simulink model "GreenCraneSimulator"  (R2021b)
settings: Solver=ode23  StartTime=0.0  StopTime=25  FixedStep=0.0001  RelTol=1e-3
values from neighbouring files (symbols this model uses):
  Annulus_area = Bore_area-Rod_area    (= 2356.19449019)    [param.m]
  beta_F = 12000e5    (= 1200000000)    [param.m]
  Bore_area = pi/4*Bore_diameter^2    (= 3318.30724035)    [param.m]
  cyl_c_end = 9e8    (= 900000000)    [param.m]
  cyl_c_visc = 1500    [param.m]
  cyl_CH_stat = 1/50    (= 0.02)    [param.m]
  cyl_F_coul = 75    [param.m]
  cyl_FH_stat = 500    [param.m]
  cyl_gamma = 250    [param.m]
  cyl_k_end = 6e9    (= 6000000000)    [param.m]
  dr_dcv = 0.7    [param.m]
  Eff_Bulk_On = 1    [param.m]
  eta_air = 0.7e-2    (= 0.007)    [param.m]
  k_cv = 15    [param.m]
  k_DCV_PA = 7.9    [param.m]
  k_DCV_PB = 7.78    [param.m]
  k_DCV_T = 7.9    [param.m]
  k_ocv = 15    [param.m]
  K_oil = 12000    [param.m]
  k_tanh = 0.005    [param.m]
  kappa_air = 1.4    [param.m]
  mu_ocv = 3    [param.m]
  OL_pa = -0.114    [param.m]
  OL_pb = 0.114    [param.m]
  p0_A = 70.5441    [param.m]
  p0_A1 = 0.99958    [param.m]
  p0_B = 1.1    [param.m]
  p_cv_fo = 1    [param.m]
  p_cv_set = 2.8    [param.m]
  p_ocv_fo = 350    [param.m]
  p_ocv_set = 150    [param.m]
  p_pc_set = 7    [param.m]
  p_R = 1.1    [param.m]
  p_S = 180    [param.m]
  patm = 1.013e5    (= 101300)    [param.m]
  Stroke = 500    [param.m]
  tau_ocv = 0.0889*0+0.055    (= 0.055)    [param.m]
  tau_pc = 0.009    [param.m]
  tCycle = 0.01    [param.m]
  UL_at = -0.05    [param.m]
  UL_bt = 0.05    [param.m]
  V_CH_A = 1.0e-03    (= 0.001)    [param.m]
  V_CH_A1 = 0.1e-03    (= 0.0001)    [param.m]
  V_CH_B = 1.25e-03    (= 0.00125)    [param.m]
  v_cyl_0 = 0    [param.m]
  wn_dcv = 30    [param.m]
  x_cyl_0 = 0.05    [param.m]
undefined symbols (not defined in the file or in its folder): DiscIntNeverNeededParam, X, Y, Z
libraries: sm_lib x25, nesl_utility x4, simulink x1
(part 2 of 2)

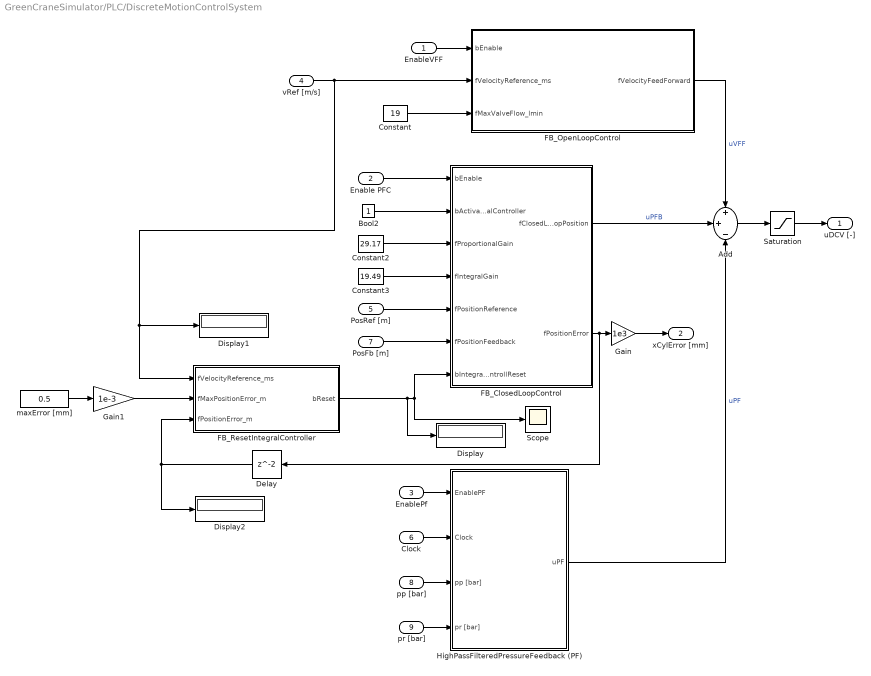
== system GreenCraneSimulator/PLC/DiscreteMotionControlSystem ==
  EnableVFF : Inport
  Enable PFC : Inport  Port=2
  EnablePf : Inport  Port=3
  vRef [m/s] : Inport  Port=4
  PosRef [m] : Inport  Port=5
  Clock : Inport  Port=6
  PosFb [m] : Inport  Port=7
  pp [bar] : Inport  Port=8
  pr [bar] : Inport  Port=9
  Add : Sum  Inputs=++-
  Bool2 : Constant  OutDataTypeStr=boolean
  Constant : Constant  Value=19
  Constant2 : Constant  Value=29.17
  Constant3 : Constant  Value=19.49
  Delay : Delay
  Display : Display
  Display1 : Display
  Display2 : Display
  FB_ClosedLoopControl : Subsystem  TreatAsAtomicUnit=on
  FB_OpenLoopControl : Subsystem  TreatAsAtomicUnit=on
  FB_ResetIntegralController : Subsystem  TreatAsAtomicUnit=on
  Gain : Gain  Gain=1e3
  Gain1 : Gain  Gain=1e-3
  HighPassFilteredPressureFeedback (PF) : Subsystem  TreatAsAtomicUnit=on  SystemSampleTime=tCycle
  Saturation : Saturate  UpperLimit=1  LowerLimit=-1
  Scope : Scope
  maxError [mm] : Constant  Value=0.5
  uDCV [-] : Outport
  xCylError [mm] : Outport  Port=2
  wires:
  Constant2/1 -> FB_ClosedLoopControl/3(fProportionalGain)
  Enable PFC/1 -> FB_ClosedLoopControl/1(bEnable)
  Constant3/1 -> FB_ClosedLoopControl/4(fIntegralGain)
  EnableVFF/1 -> FB_OpenLoopControl/1(bEnable)
  Bool2/1 -> FB_ClosedLoopControl/2(bActivateIntegralController)
  FB_ClosedLoopControl/2(fPositionError) -> Delay/1, Gain/1
  HighPassFilteredPressureFeedback (PF)/1(uPF) -> Add/3  "uPF"
  Constant/1 -> FB_OpenLoopControl/3(fMaxValveFlow_lmin)
  FB_OpenLoopControl/1(fVelocityFeedForward) -> Add/1  "uVFF"
  FB_ClosedLoopControl/1(fClosedLoopPosition) -> Add/2  "uPFB"
  PosFb [m]/1 -> FB_ClosedLoopControl/6(fPositionFeedback)
  PosRef [m]/1 -> FB_ClosedLoopControl/5(fPositionReference)
  EnablePf/1 -> HighPassFilteredPressureFeedback (PF)/1(EnablePF)
  Clock/1 -> HighPassFilteredPressureFeedback (PF)/2(Clock)
  pp [bar]/1 -> HighPassFilteredPressureFeedback (PF)/3(pp [bar])
  pr [bar]/1 -> HighPassFilteredPressureFeedback (PF)/4(pr [bar])
  Add/1 -> Saturation/1
  Gain/1 -> xCylError [mm]/1
  maxError [mm]/1 -> Gain1/1
  Saturation/1 -> uDCV [-]/1
  FB_ResetIntegralController/1(bReset) -> Display/1, FB_ClosedLoopControl/7(bIntegralControllReset), Scope/1
  Delay/1 -> FB_ResetIntegralController/3(fPositionError_m), Display2/1
  Gain1/1 -> FB_ResetIntegralController/2(fMaxPositionError_m)
  vRef [m/s]/1 -> FB_OpenLoopControl/2(fVelocityReference_ms), FB_ResetIntegralController/1(fVelocityReference_ms), Display1/1

== system GreenCraneSimulator/PLC/MotionRefSelector ==
  Auto [1] / Man [0] : Inport  OutDataTypeStr=boolean
  xCylRefGen [m] : Inport  Port=2
  vCylRefGen [m] : Inport  Port=3
  vCylJoy [m/s] : Inport  Port=4
  Data Type Conversion : DataTypeConversion  OutDataTypeStr=boolean
  Data Type Conversion1 : DataTypeConversion  OutDataTypeStr=boolean
  MATLAB Function : MATLAB Function  TreatAsAtomicUnit=on
  VFF Enable : Outport  OutDataTypeStr=boolean
  PFC Enable : Outport  Port=2  OutDataTypeStr=boolean
  vCylRef [m/s] : Outport  Port=3
  xCylRef [m] : Outport  Port=4
  wires:
  Auto [1] / Man [0]/1 -> MATLAB Function/1(AutoMode)
  vCylJoy [m/s]/1 -> MATLAB Function/4(VelRefMan)
  xCylRefGen [m]/1 -> MATLAB Function/3(PosRefAuto)
  vCylRefGen [m]/1 -> MATLAB Function/2(VelRefAuto)
  MATLAB Function/1(VelRef) -> vCylRef [m/s]/1
  MATLAB Function/2(PosRef) -> xCylRef [m]/1
  MATLAB Function/3(VFF) -> Data Type Conversion1/1
  MATLAB Function/4(PFC) -> Data Type Conversion/1
  Data Type Conversion/1 -> PFC Enable/1
  Data Type Conversion1/1 -> VFF Enable/1

== system GreenCraneSimulator/PLC/MotionReferenceTime ==
  <StartAuto> : Inport
  <StopAuto> : Inport  Port=2
  Constant : Constant
  Discrete-Time Integrator : DiscreteIntegrator  SampleTime=-1  ICPrevOutput=DiscIntNeverNeededParam  ICPrevScaledInput=DiscIntNeverNeededParam
  MATLAB Function : MATLAB Function  TreatAsAtomicUnit=on
  Time : Outport
  wires:
  <StartAuto>/1 -> MATLAB Function/1(StartClock)
  <StopAuto>/1 -> MATLAB Function/2(StopClock)
  Constant/1 -> Discrete-Time Integrator/1
  MATLAB Function/1(Time) -> Time/1
  Discrete-Time Integrator/1 -> MATLAB Function/3(Clock)

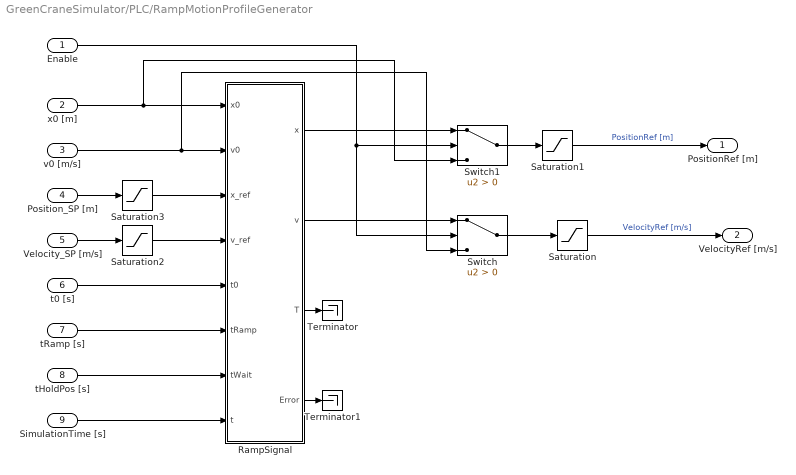
== system GreenCraneSimulator/PLC/RampMotionProfileGenerator ==
  Enable : Inport  OutDataTypeStr=boolean
  x0 [m] : Inport  Port=2  OutDataTypeStr=double
  v0 [m/s] : Inport  Port=3  OutDataTypeStr=double
  Position_SP [m] : Inport  Port=4  OutDataTypeStr=double
  "Velocity_SP [m/s] " : Inport  Port=5  OutDataTypeStr=double
  t0 [s] : Inport  Port=6  OutDataTypeStr=double
  tRamp [s] : Inport  Port=7  OutDataTypeStr=double
  tHoldPos [s] : Inport  Port=8  OutDataTypeStr=double
  SimulationTime [s] : Inport  Port=9  OutDataTypeStr=double
  RampSignal : MATLAB Function  TreatAsAtomicUnit=on
  Saturation : Saturate  UpperLimit=150  LowerLimit=-150
  Saturation1 : Saturate  UpperLimit=500  LowerLimit=0
  Saturation2 : Saturate  UpperLimit=0.120  LowerLimit=0
  Saturation3 : Saturate  LowerLimit=0
  Switch : Switch  Criteria=u2 > Threshold
  Switch1 : Switch  Criteria=u2 > Threshold
  Terminator : Terminator
  Terminator1 : Terminator
  "PositionRef [m] " : Outport  VectorParamsAs1DForOutWhenUnconnected=off
  VelocityRef [m/s] : Outport  Port=2  VectorParamsAs1DForOutWhenUnconnected=off
  wires:
  SimulationTime [s]/1 -> RampSignal/8(t)
  RampSignal/2(v) -> Switch/1
  Switch/1 -> Saturation/1
  v0 [m/s]/1 -> RampSignal/2(v0), Switch/3
  t0 [s]/1 -> RampSignal/5(t0)
  Position_SP [m]/1 -> Saturation3/1
  tHoldPos [s]/1 -> RampSignal/7(tWait)
  "Velocity_SP [m/s] "/1 -> Saturation2/1
  RampSignal/1(x) -> Switch1/1
  Enable/1 -> Switch/2, Switch1/2
  x0 [m]/1 -> Switch1/3, RampSignal/1(x0)
  Switch1/1 -> Saturation1/1
  Saturation2/1 -> RampSignal/4(v_ref)
  Saturation3/1 -> RampSignal/3(x_ref)
  tRamp [s]/1 -> RampSignal/6(tRamp)
  RampSignal/3(T) -> Terminator/1
  RampSignal/4(Error) -> Terminator1/1
  Saturation1/1 -> "PositionRef [m] "/1  "PositionRef [m]"
  Saturation/1 -> VelocityRef [m/s]/1  "VelocityRef [m/s]"

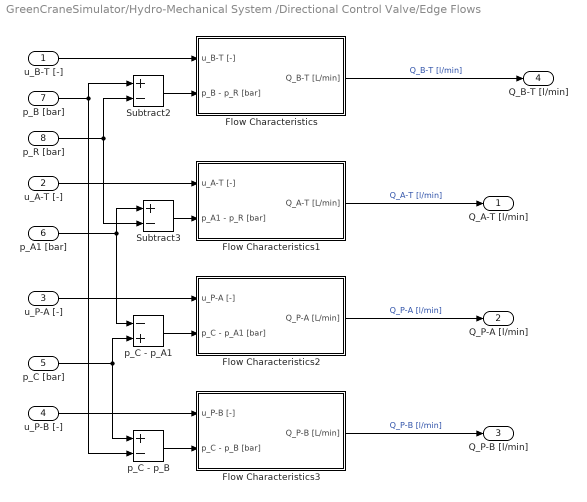
== system GreenCraneSimulator/Hydro-Mechanical System /Directional Control Valve/Edge Flows ==
  u_B-T [-] : Inport
  u_A-T [-] : Inport  Port=2
  u_P-A [-] : Inport  Port=3
  u_P-B [-] : Inport  Port=4
  p_C [bar] : Inport  Port=5
  p_A1 [bar] : Inport  Port=6
  p_B [bar] : Inport  Port=7
  p_R [bar] : Inport  Port=8
  Flow Characteristics : Subsystem
  Flow Characteristics1 : Subsystem
  Flow Characteristics2 : Subsystem
  Flow Characteristics3 : Subsystem
  Subtract2 : Sum  Inputs=+-
  Subtract3 : Sum  Inputs=+-
  p_C - p_A1 : Sum  Inputs=-+
  p_C - p_B : Sum  Inputs=+-
  Q_A-T [l/min] : Outport  VectorParamsAs1DForOutWhenUnconnected=off
  Q_P-A [l/min] : Outport  Port=2  VectorParamsAs1DForOutWhenUnconnected=off
  Q_P-B [l/min] : Outport  Port=3  VectorParamsAs1DForOutWhenUnconnected=off
  Q_B-T [l/min] : Outport  Port=4  VectorParamsAs1DForOutWhenUnconnected=off
  wires:
  p_C [bar]/1 -> p_C - p_A1/2, p_C - p_B/1
  u_A-T [-]/1 -> Flow Characteristics1/1(u_A-T [-])
  p_A1 [bar]/1 -> Subtract3/1, p_C - p_A1/1
  p_B [bar]/1 -> Subtract2/1, p_C - p_B/2
  p_C - p_B/1 -> Flow Characteristics3/2(p_C - p_B [bar])
  u_P-A [-]/1 -> Flow Characteristics2/1(u_P-A [-])
  p_C - p_A1/1 -> Flow Characteristics2/2(p_C - p_A1 [bar])
  u_P-B [-]/1 -> Flow Characteristics3/1(u_P-B [-])
  p_R [bar]/1 -> Subtract3/2, Subtract2/2
  Flow Characteristics1/1(Q_A-T [L/min]) -> Q_A-T [l/min]/1  "Q_A-T [l/min]"
  Flow Characteristics/1(Q_B-T [L/min]) -> Q_B-T [l/min]/1  "Q_B-T [l/min]"
  Flow Characteristics3/1(Q_P-B [L/min]) -> Q_P-B [l/min]/1  "Q_P-B [l/min]"
  Flow Characteristics2/1(Q_P-A [L/min]) -> Q_P-A [l/min]/1  "Q_P-A [l/min]"
  Subtract2/1 -> Flow Characteristics/2(p_B - p_R [bar])
  u_B-T [-]/1 -> Flow Characteristics/1(u_B-T [-])
  Subtract3/1 -> Flow Characteristics1/2(p_A1 - p_R [bar])

== system GreenCraneSimulator/Hydro-Mechanical System /Directional Control Valve/Edge Openings ==
  u_dcv [-] : Inport
  Edge A-T : Subsystem
  Edge B-T : Subsystem
  Edge P-A : Subsystem
  Edge P-B : Subsystem
  u_B-T [-] : Outport  VectorParamsAs1DForOutWhenUnconnected=off
  u_A-T [-] : Outport  Port=2  VectorParamsAs1DForOutWhenUnconnected=off
  u_P-A [-] : Outport  Port=3  VectorParamsAs1DForOutWhenUnconnected=off
  u_P-B [-] : Outport  Port=4  VectorParamsAs1DForOutWhenUnconnected=off
  wires:
  Edge A-T/1(u_A-T [-]) -> u_A-T [-]/1  "u_A-T [-]"
  Edge B-T/1(u_B-T [-]) -> u_B-T [-]/1  "u_B-T [-]"
  u_dcv [-]/1 -> Edge P-A/1(u_dcv [-]), Edge P-B/1(u_dcv [-]), Edge A-T/1(u_dcv [-]), Edge B-T/1(u_dcv [-])  "[-]"
  Edge P-A/1(u_P-A [-]) -> u_P-A [-]/1  "u_P-A [-]"
  Edge P-B/1(u_P-B [-]) -> u_P-B [-]/1  "u_P-B [-]"

== system GreenCraneSimulator/Hydro-Mechanical System /Directional Control Valve/Load-Sensing Pressure ==
  pB : Inport
  pA1 : Inport  Port=2
  uDCV : Inport  Port=3
  Constant : Constant  Value=0
  Switch : Switch  Criteria=u2 ~= 0
  Switch1 : Switch  Criteria=u2 > Threshold
  pLS : Outport  VectorParamsAs1DForOutWhenUnconnected=off
  wires:
  pA1/1 -> Switch1/3
  Constant/1 -> Switch/3
  Switch1/1 -> Switch/1
  Switch/1 -> pLS/1
  uDCV/1 -> Switch1/2, Switch/2
  pB/1 -> Switch1/1

== system GreenCraneSimulator/Hydro-Mechanical System /Directional Control Valve/Valve Dynamics ==
  note: 2nd order TF for
      | DCV dynamics
  u_dcv_ref [-] : Inport
  2nd order TF : TransferFcn  Denominator="[1/(wn_dcv^2) 2*dr_dcv/wn_dcv  1]"
  u_dcv [-] : Outport  VectorParamsAs1DForOutWhenUnconnected=off
  wires:
  u_dcv_ref [-]/1 -> 2nd order TF/1  "u_dcv_ref [-]"
  2nd order TF/1 -> u_dcv [-]/1  "u_dcv [-]"

== system GreenCraneSimulator/Hydro-Mechanical System /Over-Centre Valve/Capasitance ==
  Bulk Modulus : Subsystem
  Constant : Constant  Value=V_CH_A1
  Divide : Product  Inputs=*/
  "CH_A1 " : Outport  VectorParamsAs1DForOutWhenUnconnected=off
  wires:
  Bulk Modulus/1(K_oil) -> Divide/2  "[bar]"
  Constant/1 -> Divide/1  "[m^3]"
  Divide/1 -> "CH_A1 "/1

== system GreenCraneSimulator/Hydro-Mechanical System /Over-Centre Valve/Check Valve ==
  p_A [bar] : Inport
  p_A1 [bar] : Inport  Port=2
  Abs : Abs  ZeroCross=off
  Constant : Constant  Value=k_cv
  Product : Product  Inputs=****
  Saturation : Saturate  UpperLimit=1  LowerLimit=0  ZeroCross=off
  Sign : Subsystem
  Sqrt : Sqrt  SaturateOnIntegerOverflow=on
  Sum : Sum  Inputs=+-
  Sum1 : Sum  Inputs=+-
  division by p_cv_fo : Gain  Gain=1/p_cv_fo
  p_cv_set [bar] : Constant  Value=p_cv_set
  Q_cv [l/min]1 : Outport  VectorParamsAs1DForOutWhenUnconnected=off
  wires:
  p_cv_set [bar]/1 -> Sum1/2
  Sum/1 -> Abs/1, Sum1/1, Sign/1(In)  "p2-p3 [bar]"
  p_A [bar]/1 -> Sum/2
  p_A1 [bar]/1 -> Sum/1
  division by p_cv_fo/1 -> Saturation/1  "u_cv [-]"
  Sum1/1 -> division by p_cv_fo/1
  Constant/1 -> Product/1  "[l/min/bar^0.5]"
  Sqrt/1 -> Product/2  "[bar^0.5]"
  Sign/1(Out) -> Product/4
  Saturation/1 -> Product/3  "[-]"
  Abs/1 -> Sqrt/1
  Product/1 -> Q_cv [l/min]1/1

== system GreenCraneSimulator/Hydro-Mechanical System /Over-Centre Valve/Over-Centre Valve ==
  u_ocv [-] : Inport
  p_A [bar] : Inport  Port=2
  p_A1 [bar] : Inport  Port=3
  Abs : Abs  ZeroCross=off
  Product : Product  Inputs=****
  Sign : Subsystem
  Sqrt : Sqrt  SaturateOnIntegerOverflow=on
  k_ocv [l/min/bar^0.5] : Constant  Value=k_ocv
  p3-p2 : Sum  Inputs=+-
  "[l/min]" : Outport  VectorParamsAs1DForOutWhenUnconnected=off
  wires:
  k_ocv [l/min/bar^0.5]/1 -> Product/3
  p3-p2/1 -> Sign/1(In), Abs/1  "p3-p2 [bar]"
  Sqrt/1 -> Product/2  "[bar^0.5]"
  Sign/1(Out) -> Product/4
  p_A1 [bar]/1 -> p3-p2/2
  p_A [bar]/1 -> p3-p2/1
  Abs/1 -> Sqrt/1
  u_ocv [-]/1 -> Product/1  "[-]"
  Product/1 -> "[l/min]"/1

== system GreenCraneSimulator/Hydro-Mechanical System /Over-Centre Valve/Pressure Equillibrium ==
  p_B [bar] : Inport
  p_A [bar] : Inport  Port=2
  Division by p_ocv_fo [bar] : Gain  Gain=1/p_ocv_fo
  Pilot ratio [-] : Gain  Gain=mu_ocv
  Saturation : Saturate  UpperLimit=1  LowerLimit=0  ZeroCross=off
  Sum : Sum  Inputs=++-
  Valve Dynamics : TransferFcn  Denominator=[tau_ocv 1]
  p_ocv_set [bar] : Constant  Value=p_ocv_set
  u_ocv [-] : Outport  VectorParamsAs1DForOutWhenUnconnected=off
  wires:
  Sum/1 -> Division by p_ocv_fo [bar]/1  "[bar]"
  Pilot ratio [-]/1 -> Sum/1
  p_ocv_set [bar]/1 -> Sum/3
  p_B [bar]/1 -> Pilot ratio [-]/1
  p_A [bar]/1 -> Sum/2
  Valve Dynamics/1 -> u_ocv [-]/1  "[-]"
  Division by p_ocv_fo [bar]/1 -> Saturation/1  "u_ocv_ref [-]"
  Saturation/1 -> Valve Dynamics/1

== system GreenCraneSimulator/Hydro-Mechanical System /Subsystem/CH Bore Side ==
  x [m] : Inport
  Bulk Modulus : Subsystem
  Constant4 : Constant  Value=V_CH_A
  Divide2 : Product  Inputs=*/
  Gain1 : Gain  Gain=Bore_area
  Gain2 : Gain  Gain=1/(10)^9
  Gain3 : Gain  Gain=1000
  Scope : Scope
  Sum3 : Sum
  CH_A : Outport  VectorParamsAs1DForOutWhenUnconnected=off
  wires:
  Sum3/1 -> Divide2/1  "[m^3]"
  x [m]/1 -> Gain3/1
  Constant4/1 -> Sum3/1  "[m^3]"
  Gain1/1 -> Gain2/1  "[mm^3]"
  Gain3/1 -> Gain1/1  "[mm]"
  Gain2/1 -> Scope/1, Sum3/2  "[m^3]"
  Divide2/1 -> CH_A/1
  Bulk Modulus/1(K_oil) -> Divide2/2  "[bar]"

== system GreenCraneSimulator/Hydro-Mechanical System /Subsystem/CH Rod Side ==
  x [m] : Inport
  Bulk Modulus : Subsystem
  Constant1 : Constant  Value=Stroke
  Constant4 : Constant  Value=V_CH_B
  Divide2 : Product  Inputs=*/
  Gain1 : Gain  Gain=Annulus_area
  Gain2 : Gain  Gain=1/(10)^9
  Gain4 : Gain  Gain=1000
  Scope : Scope
  Sum2 : Sum  Inputs=+-
  Sum3 : Sum
  CH_B : Outport  VectorParamsAs1DForOutWhenUnconnected=off
  wires:
  Sum3/1 -> Divide2/1  "[m^3]"
  Constant1/1 -> Sum2/1  "[mm]"
  x [m]/1 -> Gain4/1
  Sum2/1 -> Gain1/1
  Constant4/1 -> Sum3/1  "[m^3]"
  Gain1/1 -> Gain2/1  "[mm^3]"
  Gain4/1 -> Sum2/2  "[mm]"
  Gain2/1 -> Sum3/2, Scope/1  "[m^3]"
  Divide2/1 -> CH_B/1
  Bulk Modulus/1(K_oil) -> Divide2/2

== system GreenCraneSimulator/Hydro-Mechanical System /Subsystem/Cylinder forces ==
  v_cyl [m/s] : Inport
  F_hyd [N] : Inport  Port=2
  x _cyl [m] : Inport  Port=3
  Add : Sum  Inputs=+-+-
  Lower Stroke Limit : Subsystem
  Stribeck Friction1 : Subsystem
  Upper Stroke Limit : Subsystem
  F_piston [N] : Outport  VectorParamsAs1DForOutWhenUnconnected=off
  wires:
  Lower Stroke Limit/1(F_cyl_contact [N]) -> Add/3
  Upper Stroke Limit/1(F_cyl_contact [N]) -> Add/2
  x _cyl [m]/1 -> Upper Stroke Limit/1(x_cyl [m]), Lower Stroke Limit/1(x_cyl [m])
  Add/1 -> F_piston [N]/1  "Bm_Cyl_F"
  v_cyl [m/s]/1 -> Stribeck Friction1/1(v_cyl [m/s]), Lower Stroke Limit/2(v_cyl [m]), Upper Stroke Limit/2(v_cyl [m/s])
  Stribeck Friction1/1(F [N]) -> Add/4
  F_hyd [N]/1 -> Add/1

== system GreenCraneSimulator/PC | Ubuntu | ROS2/Green Crane | Visualizer /Setup ==
  Mechanism Configuration1 : sm_lib/Utilities/Mechanism Configuration  UniformGravity=Constant  GravityVector=[0 0 -9.80665]  GravityUnits=m/s^2  LinearizationDelta=0.001  JointModeTransitionNonlinearIterations=2
  Solver Configuration : nesl_utility/Solver Configuration  PhysicalDomain=network_engine_domain  SubClassName=solver  LeftPortType=input  RightPortType=generic  Tones=[]  Harmonics=[]  SimulateNoise=off  Profile=off  UseLocalSampling=off  EnableSwitchedLinearOptims=on  FrequencyDomain=off  UseCCode=off  RelTol=0.001  AbsTol=1e-06  MinStep=1e-09  ToWorkspace=off  RevertToSquareIcSolve=off  NumHomotopyIterations=100  PhasorMode=off  PhasorModeNumHarmonics=1  DoDC=off  ResidualTolerance=1e-09  UseLocalSolver=off  LocalSolverChoice=NE_BACKWARD_EULER_ADVANCER  LocalSolverSampleTime=0.001  DoFixedCost=off  MaxNonlinIter=3  MaxModeIter=2  ComputeImpulses=off  ImpulseIterations=2  LinearAlgebra=Sparse  EquationFormulation=NE_TIME_EF  DelaysMemoryBudget=1024  AutomaticFiltering=on  FilteringTimeConstant=0.001  PartitionStorageMethod=AS_NEEDED  PartitionMemoryBudget=1024  PartitionMethod=FAST
      settings: SourceProductBaseCode=PW,SS
  World Frame : sm_lib/Frames and Transforms/World Frame
  Origin : PMIOPort  Side=Right
  connections:
  Solver Configuration/RConn1 -- World Frame/RConn1 -- Mechanism Configuration1/RConn1 -- Origin/RConn1

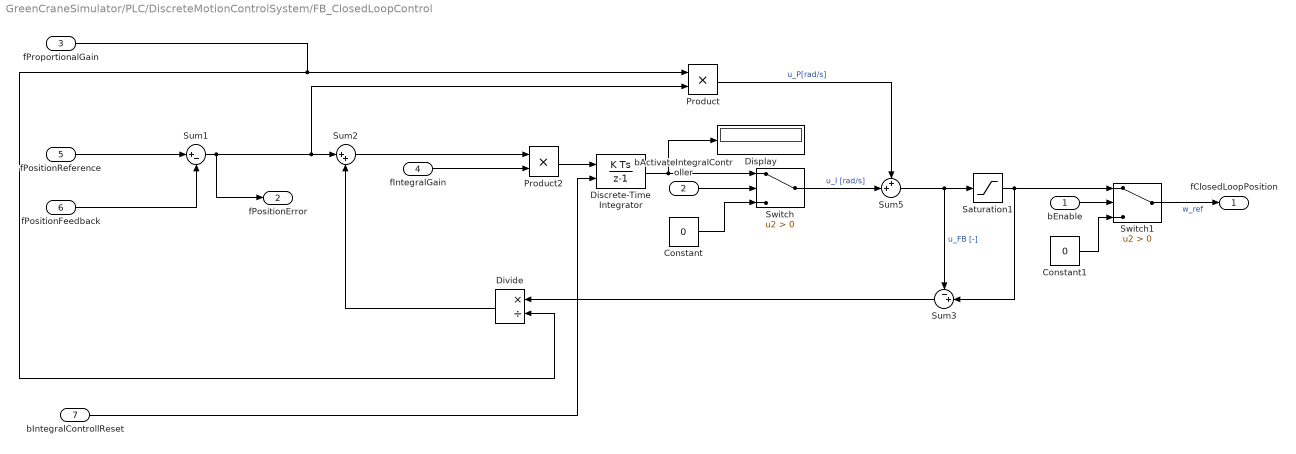
== system GreenCraneSimulator/PLC/DiscreteMotionControlSystem/FB_ClosedLoopControl ==
  bEnable : Inport  OutDataTypeStr=boolean
  bActivateIntegralController : Inport  Port=2  OutDataTypeStr=boolean
  fProportionalGain : Inport  Port=3
  fIntegralGain : Inport  Port=4
  fPositionReference : Inport  Port=5
  fPositionFeedback : Inport  Port=6
  bIntegralControllReset : Inport  Port=7  OutDataTypeStr=boolean
  Constant : Constant  Value=0
  Constant1 : Constant  Value=0
  Discrete-Time Integrator : DiscreteIntegrator  ExternalReset=sampled level  SampleTime=-1  LimitOutput=on  UpperSaturationLimit=1  LowerSaturationLimit=-1  ICPrevOutput=DiscIntNeverNeededParam  ICPrevScaledInput=DiscIntNeverNeededParam
  Display : Display
  Divide : Product  Inputs=*/
  Product : Product
  Product2 : Product
  Saturation1 : Saturate  UpperLimit=1  LowerLimit=-1
  Sum1 : Sum  Inputs=|+-
  Sum2 : Sum  Inputs=|++
  Sum3 : Sum  Inputs=-+|
  Sum5 : Sum  Inputs=++|
  Switch : Switch  Criteria=u2 > Threshold
  Switch1 : Switch  Criteria=u2 > Threshold
  fClosedLoopPosition : Outport  VectorParamsAs1DForOutWhenUnconnected=off
  fPositionError : Outport  Port=2  VectorParamsAs1DForOutWhenUnconnected=off
  wires:
  fPositionFeedback/1 -> Sum1/2
  Sum2/1 -> Product2/1
  Divide/1 -> Sum2/2
  fProportionalGain/1 -> Product/1, Divide/2
  fIntegralGain/1 -> Product2/2
  bActivateIntegralController/1 -> Switch/2
  Constant/1 -> Switch/3
  fPositionReference/1 -> Sum1/1
  Sum5/1 -> Sum3/1, Saturation1/1  "u_FB [-]"
  Sum3/1 -> Divide/1
  Switch1/1 -> fClosedLoopPosition/1  "w_ref"
  Constant1/1 -> Switch1/3
  bEnable/1 -> Switch1/2
  Saturation1/1 -> Switch1/1, Sum3/2
  Product/1 -> Sum5/1  "u_P[rad/s]"
  Switch/1 -> Sum5/2  "u_I [rad/s]"
  Product2/1 -> Discrete-Time Integrator/1
  bIntegralControllReset/1 -> Discrete-Time Integrator/2
  Discrete-Time Integrator/1 -> Display/1, Switch/1
  Sum1/1 -> fPositionError/1, Product/2, Sum2/1

== system GreenCraneSimulator/PLC/DiscreteMotionControlSystem/FB_OpenLoopControl ==
  bEnable : Inport  OutDataTypeStr=boolean
  fVelocityReference_ms : Inport  Port=2
  fMaxValveFlow_lmin : Inport  Port=3
  Annnulus_Area : Constant  Value=0.0023562
  Bore_Area : Constant  Value=0.0033183
  Constant : Constant  Value=0
  Divide2 : Product  Inputs=*/
  Gain1 : Gain  Gain=60000
  Product1 : Product
  Product3 : Product
  Switch1 : Switch  Criteria=u2 > Threshold
  Switch2 : Switch
  fVelocityFeedForward : Outport  VectorParamsAs1DForOutWhenUnconnected=off
  wires:
  Annnulus_Area/1 -> Product3/2  "[m^2]"
  Switch2/1 -> Gain1/1  "Q_ref [m^3/s]"
  Product1/1 -> Switch2/1
  fVelocityReference_ms/1 -> Product3/1, Product1/2, Switch2/2
  fMaxValveFlow_lmin/1 -> Divide2/2  "Qmax [l/min]"
  Bore_Area/1 -> Product1/1  "[m^2]"
  Gain1/1 -> Divide2/1  "Q_ref [L/min]"
  Product3/1 -> Switch2/3
  Constant/1 -> Switch1/3
  Divide2/1 -> Switch1/1
  bEnable/1 -> Switch1/2
  Switch1/1 -> fVelocityFeedForward/1

== system GreenCraneSimulator/PLC/DiscreteMotionControlSystem/FB_ResetIntegralController ==
  fVelocityReference_ms : Inport
  fMaxPositionError_m : Inport  Port=2
  fPositionError_m : Inport  Port=3
  Data Type Conversion : DataTypeConversion  OutDataTypeStr=boolean
  ResetIntegralController : MATLAB Function  TreatAsAtomicUnit=on
  bReset : Outport  OutDataTypeStr=boolean
  wires:
  fMaxPositionError_m/1 -> ResetIntegralController/2(exCylMax)
  fVelocityReference_ms/1 -> ResetIntegralController/1(vRef)
  ResetIntegralController/1(Reset) -> Data Type Conversion/1
  fPositionError_m/1 -> ResetIntegralController/3(exCyl)
  Data Type Conversion/1 -> bReset/1

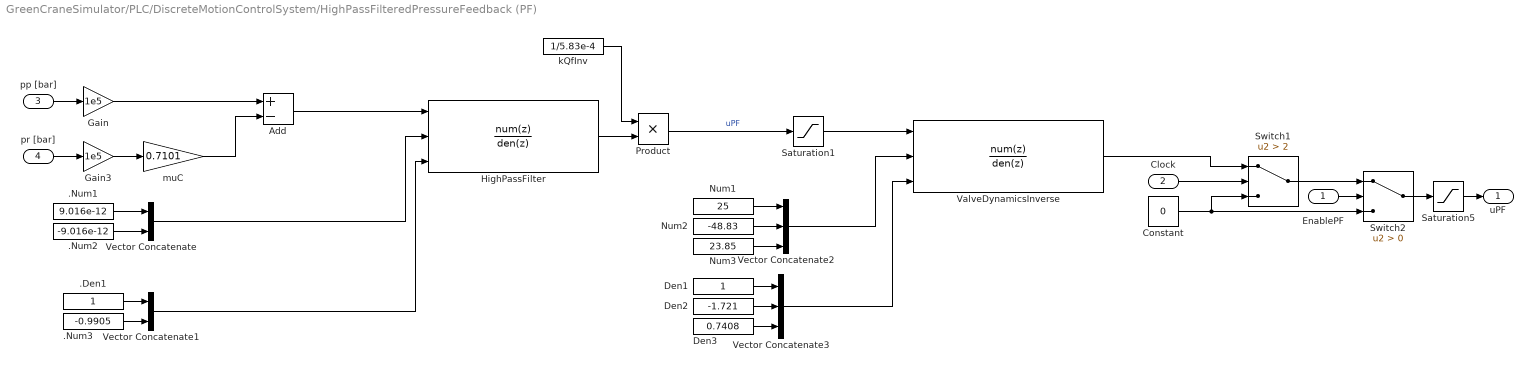
== system GreenCraneSimulator/PLC/DiscreteMotionControlSystem/HighPassFilteredPressureFeedback (PF) ==
  EnablePF : Inport  OutDataTypeStr=boolean
  Clock : Inport  Port=2
  pp [bar] : Inport  Port=3
  pr [bar] : Inport  Port=4
  .Den1 : Constant
  .Num1 : Constant  Value=9.016e-12
  .Num2 : Constant  Value=-9.016e-12
  .Num3 : Constant  Value=-0.9905
  Add : Sum  Inputs=+-
  Constant : Constant  Value=0
  Den1 : Constant
  Den2 : Constant  Value=-1.721
  Den3 : Constant  Value=0.7408
  Gain : Gain  Gain=1e5
  Gain3 : Gain  Gain=1e5
  HighPassFilter : DiscreteTransferFcn  NumeratorSource=Input port  Numerator=[3.786e-11 -3.786e-11]  DenominatorSource=Input port  Denominator=[1 -0.9954]  a0EqualsOne=on
      settings: InputPortMap=u0,p1,p3
  Num1 : Constant  Value=25
  Num2 : Constant  Value=-48.83
  Num3 : Constant  Value=23.85
  Product : Product
  Saturation1 : Saturate  UpperLimit=1  LowerLimit=-1
  Saturation5 : Saturate  UpperLimit=1  LowerLimit=-1
  Switch1 : Switch  Criteria=u2 > Threshold  Threshold=2
  Switch2 : Switch  Criteria=u2 > Threshold
  ValveDynamicsInverse : DiscreteTransferFcn  NumeratorSource=Input port  Numerator=[25 -48.83 23.85]  DenominatorSource=Input port  Denominator=[1 -1.721 0.7408]  a0EqualsOne=on
      settings: InputPortMap=u0,p1,p3
  Vector Concatenate : Concatenate
  Vector Concatenate1 : Concatenate
  Vector Concatenate2 : Concatenate  NumInputs=3
  Vector Concatenate3 : Concatenate  NumInputs=3
  kQfInv : Constant  Value=1/5.83e-4
  muC : Gain  Gain=0.7101
  uPF : Outport  VectorParamsAs1DForOutWhenUnconnected=off
  wires:
  pr [bar]/1 -> Gain3/1
  pp [bar]/1 -> Gain/1
  Add/1 -> HighPassFilter/1
  Gain/1 -> Add/1
  HighPassFilter/1 -> Product/2
  Constant/1 -> Switch1/3, Switch2/3
  Gain3/1 -> muC/1
  Vector Concatenate/1 -> HighPassFilter/2
  Vector Concatenate1/1 -> HighPassFilter/3
  .Num1/1 -> Vector Concatenate/1
  .Num2/1 -> Vector Concatenate/2
  .Den1/1 -> Vector Concatenate1/1
  .Num3/1 -> Vector Concatenate1/2
  Switch2/1 -> Saturation5/1
  Switch1/1 -> Switch2/1
  EnablePF/1 -> Switch2/2
  Saturation5/1 -> uPF/1
  Vector Concatenate2/1 -> ValveDynamicsInverse/2
  Vector Concatenate3/1 -> ValveDynamicsInverse/3
  Den1/1 -> Vector Concatenate3/1
  Den2/1 -> Vector Concatenate3/2
  Den3/1 -> Vector Concatenate3/3
  ValveDynamicsInverse/1 -> Switch1/1
  kQfInv/1 -> Product/1
  muC/1 -> Add/2
  Num1/1 -> Vector Concatenate2/1
  Num2/1 -> Vector Concatenate2/2
  Num3/1 -> Vector Concatenate2/3
  Saturation1/1 -> ValveDynamicsInverse/1
  Product/1 -> Saturation1/1  "uPF"
  Clock/1 -> Switch1/2

== system GreenCraneSimulator/Hydro-Mechanical System /Directional Control Valve/Edge Flows/Flow Characteristics ==
  u_B-T [-] : Inport
  p_B - p_R [bar] : Inport  Port=2
  Abs : Abs
  Constant : Constant  Value=k_DCV_T
  Product6 : Product  Inputs=4  RndMeth=Zero
  Sign : Subsystem
  Sqrt7 : Sqrt  SaturateOnIntegerOverflow=on
  Q_B-T [L/min] : Outport  VectorParamsAs1DForOutWhenUnconnected=off
  wires:
  Sqrt7/1 -> Product6/3  "[bar]^0.5"
  Product6/1 -> Q_B-T [L/min]/1  "[L/min]"
  p_B - p_R [bar]/1 -> Sign/1(In), Abs/1  "[bar]"
  Abs/1 -> Sqrt7/1
  u_B-T [-]/1 -> Product6/2  "[-]"
  Constant/1 -> Product6/1  "[L/min*bar^0.5]"
  Sign/1(Out) -> Product6/4

== system GreenCraneSimulator/Hydro-Mechanical System /Directional Control Valve/Edge Flows/Flow Characteristics1 ==
  u_A-T [-] : Inport
  p_A1 - p_R [bar] : Inport  Port=2
  Abs : Abs
  Constant : Constant  Value=k_DCV_T
  Product6 : Product  Inputs=4  RndMeth=Zero
  Sign : Subsystem
  Sqrt7 : Sqrt  SaturateOnIntegerOverflow=on
  Q_A-T [L/min] : Outport  VectorParamsAs1DForOutWhenUnconnected=off
  wires:
  Sqrt7/1 -> Product6/3  "[bar]^0.5"
  Product6/1 -> Q_A-T [L/min]/1  "[L/min]"
  p_A1 - p_R [bar]/1 -> Sign/1(In), Abs/1  "[bar]"
  Abs/1 -> Sqrt7/1
  u_A-T [-]/1 -> Product6/2  "[-]"
  Sign/1(Out) -> Product6/4
  Constant/1 -> Product6/1  "[L/min*bar^0.5]"

== system GreenCraneSimulator/Hydro-Mechanical System /Directional Control Valve/Edge Flows/Flow Characteristics2 ==
  u_P-A [-] : Inport
  p_C - p_A1 [bar] : Inport  Port=2
  Abs : Abs
  Constant : Constant  Value=k_DCV_PA
  Product6 : Product  Inputs=4  RndMeth=Zero
  Sign : Subsystem
  Sqrt7 : Sqrt  SaturateOnIntegerOverflow=on
  Q_P-A [L/min] : Outport  VectorParamsAs1DForOutWhenUnconnected=off
  wires:
  Sqrt7/1 -> Product6/3  "[bar]^0.5"
  Product6/1 -> Q_P-A [L/min]/1  "[L/min]"
  p_C - p_A1 [bar]/1 -> Sign/1(In), Abs/1  "[bar]"
  Abs/1 -> Sqrt7/1
  u_P-A [-]/1 -> Product6/2  "[-]"
  Sign/1(Out) -> Product6/4
  Constant/1 -> Product6/1  "[L/min*bar^0.5]"

== system GreenCraneSimulator/Hydro-Mechanical System /Directional Control Valve/Edge Flows/Flow Characteristics3 ==
  u_P-B [-] : Inport
  p_C - p_B [bar] : Inport  Port=2
  Abs : Abs
  Constant : Constant  Value=k_DCV_PB
  Product6 : Product  Inputs=4  RndMeth=Zero
  Sign : Subsystem
  Sqrt7 : Sqrt  SaturateOnIntegerOverflow=on
  Q_P-B [L/min] : Outport  VectorParamsAs1DForOutWhenUnconnected=off
  wires:
  Sqrt7/1 -> Product6/3  "[bar]^0.5"
  Product6/1 -> Q_P-B [L/min]/1  "[L/min]"
  p_C - p_B [bar]/1 -> Sign/1(In), Abs/1  "[bar]"
  Abs/1 -> Sqrt7/1
  u_P-B [-]/1 -> Product6/2  "[-]"
  Sign/1(Out) -> Product6/4
  Constant/1 -> Product6/1  "[L/min*bar^0.5]"

== system GreenCraneSimulator/Hydro-Mechanical System /Directional Control Valve/Edge Openings/Edge A-T ==
  u_dcv [-] : Inport
  MATLAB Function1 : MATLAB Function  TreatAsAtomicUnit=on
  u_A-T [-] : Outport  VectorParamsAs1DForOutWhenUnconnected=off
  wires:
  MATLAB Function1/1(u_AT) -> u_A-T [-]/1
  u_dcv [-]/1 -> MATLAB Function1/1(u_dcv)

== system GreenCraneSimulator/Hydro-Mechanical System /Directional Control Valve/Edge Openings/Edge B-T ==
  u_dcv [-] : Inport
  MATLAB Function : MATLAB Function  TreatAsAtomicUnit=on
  u_B-T [-] : Outport  VectorParamsAs1DForOutWhenUnconnected=off
  wires:
  u_dcv [-]/1 -> MATLAB Function/1(u_dcv)
  MATLAB Function/1(u_BT) -> u_B-T [-]/1

== system GreenCraneSimulator/Hydro-Mechanical System /Directional Control Valve/Edge Openings/Edge P-A ==
  u_dcv [-] : Inport
  MATLAB Function1 : MATLAB Function  TreatAsAtomicUnit=on
  u_P-A [-] : Outport  VectorParamsAs1DForOutWhenUnconnected=off
  wires:
  u_dcv [-]/1 -> MATLAB Function1/1(u_dcv)
  MATLAB Function1/1(u_PA) -> u_P-A [-]/1

== system GreenCraneSimulator/Hydro-Mechanical System /Directional Control Valve/Edge Openings/Edge P-B ==
  u_dcv [-] : Inport
  MATLAB Function1 : MATLAB Function  TreatAsAtomicUnit=on
  u_P-B [-] : Outport  VectorParamsAs1DForOutWhenUnconnected=off
  wires:
  u_dcv [-]/1 -> MATLAB Function1/1(u_dcv)
  MATLAB Function1/1(u_PB) -> u_P-B [-]/1

== system GreenCraneSimulator/Hydro-Mechanical System /Over-Centre Valve/Capasitance/Bulk Modulus ==
  Bulk/Volume : Constant  Value=K_oil
  Eff_Bulk_On : Constant  Value=Eff_Bulk_On
  Effective Bulk Modulus : Subsystem
  Switch : Switch  Criteria=u2 > Threshold
  K_oil : Outport  VectorParamsAs1DForOutWhenUnconnected=off
  wires:
  Bulk/Volume/1 -> Switch/3  "[bar]"
  Switch/1 -> K_oil/1
  Eff_Bulk_On/1 -> Switch/2
  Effective Bulk Modulus/1(K_oil_eff) -> Switch/1  "[bar]"

== system GreenCraneSimulator/Hydro-Mechanical System /Over-Centre Valve/Check Valve/Sign ==
  In : Inport
  Gain2 : Gain  Gain=1/k_tanh
  Trigonometric Function : Trigonometry  Operator=tanh
  Out : Outport  VectorParamsAs1DForOutWhenUnconnected=off
  wires:
  In/1 -> Gain2/1
  Gain2/1 -> Trigonometric Function/1
  Trigonometric Function/1 -> Out/1  "[-]"

== system GreenCraneSimulator/Hydro-Mechanical System /Over-Centre Valve/Over-Centre Valve/Sign ==
  In : Inport
  Gain2 : Gain  Gain=1/k_tanh
  Trigonometric Function : Trigonometry  Operator=tanh
  Out : Outport  VectorParamsAs1DForOutWhenUnconnected=off
  wires:
  In/1 -> Gain2/1
  Gain2/1 -> Trigonometric Function/1
  Trigonometric Function/1 -> Out/1  "[-]"

== system GreenCraneSimulator/Hydro-Mechanical System /Subsystem/CH Bore Side/Bulk Modulus ==
  Bulk/Volume : Constant  Value=K_oil
  Eff_Bulk_On : Constant  Value=Eff_Bulk_On
  Effective Bulk Modulus : Subsystem
  Switch : Switch  Criteria=u2 > Threshold
  K_oil : Outport  VectorParamsAs1DForOutWhenUnconnected=off
  wires:
  Bulk/Volume/1 -> Switch/3  "[bar]"
  Switch/1 -> K_oil/1
  Eff_Bulk_On/1 -> Switch/2
  Effective Bulk Modulus/1(K_oil_eff) -> Switch/1  "[bar]"

== system GreenCraneSimulator/Hydro-Mechanical System /Subsystem/CH Rod Side/Bulk Modulus ==
  Bulk/Volume : Constant  Value=K_oil
  Eff_Bulk_On : Constant  Value=Eff_Bulk_On
  Effective Bulk Modulus : Subsystem
  Switch : Switch  Criteria=u2 > Threshold
  K_oil : Outport  VectorParamsAs1DForOutWhenUnconnected=off
  wires:
  Bulk/Volume/1 -> Switch/3  "[bar]"
  Switch/1 -> K_oil/1
  Eff_Bulk_On/1 -> Switch/2
  Effective Bulk Modulus/1(K_oil_eff) -> Switch/1  "[bar]"

== system GreenCraneSimulator/Hydro-Mechanical System /Subsystem/Cylinder forces/Lower Stroke Limit ==
  x_cyl [m] : Inport
  v_cyl [m] : Inport  Port=2
  Abs : Abs
  Add1 : Sum
  Constant : Constant  Value=0
  Constant1 : Constant  Value=0
  End stroke spring coeff : Constant  Value=cyl_k_end
  End stroke viscous coeff : Constant  Value=cyl_c_end
  Gain : Gain  Gain=-1
  Saturation : Saturate  UpperLimit=0  LowerLimit=-inf
  Switch : Switch  Criteria=u2 > Threshold
  Switch1 : Switch  Criteria=u2 > Threshold
  mult : Product  Inputs=**
  mult1 : Product  Inputs=**
  F_cyl_contact [N] : Outport  VectorParamsAs1DForOutWhenUnconnected=off
  wires:
  Add1/1 -> F_cyl_contact [N]/1
  mult1/1 -> Saturation/1
  mult/1 -> Add1/1
  Switch1/1 -> Gain/1
  Abs/1 -> mult/2
  Switch/1 -> mult/1
  x_cyl [m]/1 -> Switch1/2, Abs/1, Switch/2
  Constant/1 -> Switch/1
  End stroke spring coeff/1 -> Switch/3
  End stroke viscous coeff/1 -> Switch1/3
  Constant1/1 -> Switch1/1
  Gain/1 -> mult1/1
  v_cyl [m]/1 -> mult1/2
  Saturation/1 -> Add1/2

== system GreenCraneSimulator/Hydro-Mechanical System /Subsystem/Cylinder forces/Stribeck Friction1 ==
  v_cyl [m/s] : Inport
  Mux : Mux  Inputs=6
  Stribeck Curve : Fcn  Expr=u(1)*u(2)+tanh(u(1)*u(3))*(u(4)+u(5)*exp(-(u(1)*tanh(u(1)*u(3)))/u(6)))
  "coefficient of viscous friction " : Constant  Value=cyl_c_visc
  coulomb friction : Constant  Value=cyl_F_coul
  friction force approximation constant : Constant  Value=cyl_gamma
  friction time constant : Constant  Value=cyl_CH_stat
  static friction : Constant  Value=cyl_FH_stat
  F [N] : Outport  VectorParamsAs1DForOutWhenUnconnected=off
  wires:
  v_cyl [m/s]/1 -> Mux/1
  Stribeck Curve/1 -> F [N]/1
  friction time constant/1 -> Mux/6
  static friction/1 -> Mux/5
  coulomb friction/1 -> Mux/4
  friction force approximation constant/1 -> Mux/3
  "coefficient of viscous friction "/1 -> Mux/2
  Mux/1 -> Stribeck Curve/1

== system GreenCraneSimulator/Hydro-Mechanical System /Subsystem/Cylinder forces/Upper Stroke Limit ==
  x_cyl [m] : Inport
  v_cyl [m/s] : Inport  Port=2
  Add : Sum  Inputs=|+-
  Add1 : Sum
  Constant : Constant  Value=0
  Constant1 : Constant  Value=0
  End stroke spring coeff : Constant  Value=cyl_k_end
  End stroke viscous coeff : Constant  Value=cyl_c_end
  Gain : Gain  Gain=1/1000
  Saturation : Saturate  UpperLimit=inf  LowerLimit=0
  Stroke Length : Constant  Value=Stroke
  Switch : Switch  Criteria=u2 > Threshold  Threshold=Stroke/1000
  Switch1 : Switch  Criteria=u2 > Threshold  Threshold=Stroke/1000
  mult : Product  Inputs=**
  mult1 : Product  Inputs=**
  F_cyl_contact [N] : Outport  VectorParamsAs1DForOutWhenUnconnected=off
  wires:
  x_cyl [m]/1 -> Add/1, Switch1/2, Switch/2
  End stroke spring coeff/1 -> Switch/1
  Constant/1 -> Switch/3
  Stroke Length/1 -> Gain/1
  Switch/1 -> mult/1
  Add/1 -> mult/2
  End stroke viscous coeff/1 -> Switch1/1
  Constant1/1 -> Switch1/3
  Switch1/1 -> mult1/1
  mult/1 -> Add1/1
  mult1/1 -> Saturation/1
  Add1/1 -> F_cyl_contact [N]/1
  v_cyl [m/s]/1 -> mult1/2
  Saturation/1 -> Add1/2
  Gain/1 -> Add/2  "[m]"

== system GreenCraneSimulator/Hydro-Mechanical System /Directional Control Valve/Edge Flows/Flow Characteristics/Sign ==
  In : Inport
  Gain2 : Gain  Gain=1/k_tanh
  Trigonometric Function : Trigonometry  Operator=tanh
  Out : Outport  VectorParamsAs1DForOutWhenUnconnected=off
  wires:
  In/1 -> Gain2/1
  Gain2/1 -> Trigonometric Function/1
  Trigonometric Function/1 -> Out/1  "[-]"

== system GreenCraneSimulator/Hydro-Mechanical System /Directional Control Valve/Edge Flows/Flow Characteristics1/Sign ==
  In : Inport
  Gain2 : Gain  Gain=1/k_tanh
  Trigonometric Function : Trigonometry  Operator=tanh
  Out : Outport  VectorParamsAs1DForOutWhenUnconnected=off
  wires:
  In/1 -> Gain2/1
  Gain2/1 -> Trigonometric Function/1
  Trigonometric Function/1 -> Out/1  "[-]"

== system GreenCraneSimulator/Hydro-Mechanical System /Directional Control Valve/Edge Flows/Flow Characteristics2/Sign ==
  In : Inport
  Gain2 : Gain  Gain=1/k_tanh
  Trigonometric Function : Trigonometry  Operator=tanh
  Out : Outport  VectorParamsAs1DForOutWhenUnconnected=off
  wires:
  In/1 -> Gain2/1
  Gain2/1 -> Trigonometric Function/1
  Trigonometric Function/1 -> Out/1  "[-]"

== system GreenCraneSimulator/Hydro-Mechanical System /Directional Control Valve/Edge Flows/Flow Characteristics3/Sign ==
  In : Inport
  Gain2 : Gain  Gain=1/k_tanh
  Trigonometric Function : Trigonometry  Operator=tanh
  Out : Outport  VectorParamsAs1DForOutWhenUnconnected=off
  wires:
  In/1 -> Gain2/1
  Gain2/1 -> Trigonometric Function/1
  Trigonometric Function/1 -> Out/1  "[-]"

== system GreenCraneSimulator/Hydro-Mechanical System /Over-Centre Valve/Capasitance/Bulk Modulus/Effective Bulk Modulus ==
  2 : Scope
  MATLAB Function : MATLAB Function  TreatAsAtomicUnit=on
  K_oil_eff : Outport  VectorParamsAs1DForOutWhenUnconnected=off
  wires:
  MATLAB Function/1(K_oil_eff) -> K_oil_eff/1, 2/1
  [p_A1] -> MATLAB Function/1(p)

== system GreenCraneSimulator/Hydro-Mechanical System /Subsystem/CH Bore Side/Bulk Modulus/Effective Bulk Modulus ==
  MATLAB Function : MATLAB Function  TreatAsAtomicUnit=on
  K_oil_eff : Outport  VectorParamsAs1DForOutWhenUnconnected=off
  wires:
  MATLAB Function/1(K_oil_eff) -> K_oil_eff/1
  [p_A] -> MATLAB Function/1(p)

== system GreenCraneSimulator/Hydro-Mechanical System /Subsystem/CH Rod Side/Bulk Modulus/Effective Bulk Modulus ==
  MATLAB Function : MATLAB Function  TreatAsAtomicUnit=on
  K_oil_eff : Outport  VectorParamsAs1DForOutWhenUnconnected=off
  wires:
  MATLAB Function/1(K_oil_eff) -> K_oil_eff/1
  [p_B] -> MATLAB Function/1(p)

== matlab function GreenCraneSimulator/Hydro-Mechanical System /Directional Control Valve/Edge Openings/Edge A-T/MATLAB Function1 ==
  data: u_dcv input; u_AT output; OL_pa parameter; OL_pb parameter; UL_at parameter; UL_bt parameter
function u_AT = fcn(u_dcv,OL_pa, OL_pb, UL_at, UL_bt)

u_AT = 0;

if u_dcv <= UL_at
 u_AT = 0;
 
elseif u_dcv > UL_at   && u_dcv < 2*OL_pb
 u_AT= ((u_dcv-UL_at)*OL_pb)/((1-OL_pb)*(-UL_at+2*OL_pb));
 
elseif 2*OL_pb <= u_dcv
  u_AT= (u_dcv-OL_pb)/(1-OL_pb);
end

== matlab function GreenCraneSimulator/PLC/DiscreteMotionControlSystem/FB_ResetIntegralController/ResetIntegralController ==
  data: vRef input; exCylMax input; Reset output; exCyl input
function Reset = fcn(vRef, exCylMax, exCyl)

if abs(vRef) > 0 || abs(exCyl) > exCylMax
Reset = 0;
else 
Reset = 1;
end

== matlab function GreenCraneSimulator/Hydro-Mechanical System /Directional Control Valve/Edge Openings/Edge B-T/MATLAB Function ==
  data: u_dcv input; u_BT output; OL_pa parameter; OL_pb parameter; UL_at parameter; UL_bt parameter
function u_BT = fcn(u_dcv,OL_pa, OL_pb, UL_at, UL_bt)

  u_BT = 0;

if UL_bt <=  u_dcv 
 u_BT = 0;
 
elseif 2*OL_pa < u_dcv && u_dcv < UL_bt
 u_BT= ((u_dcv-UL_bt)*OL_pa)/((1+OL_pa)*(UL_bt-2*OL_pa));
 
elseif u_dcv <=  2*OL_pa
  u_BT= -(u_dcv-OL_pa)/(1+OL_pa);
end

== matlab function GreenCraneSimulator/PLC/MotionReferenceTime/MATLAB Function ==
  data: StartClock input; StopClock input; Time output; Clock input
function Time = fcn(StartClock, StopClock, Clock)

if StartClock == 1 && ~StopClock
Time = Clock;
else
Time = 0.0;     
end

== matlab function GreenCraneSimulator/PLC/CylinderDiscplacementToBoomAngle ==
  data: thetaBoom output; xCyl input
function thetaBoom  = fcn(xCyl)

%% Geomtry Constants
ABx = 0.427;
ABy = 1.057;
ACx = 0.49484;
ACy = 0.133;

AB = sqrt(abs(ABx)^2 + abs(ABy)^2);
AC = sqrt(abs(ACx)^2 + abs(ACy)^2);

BC = 0.77222 + xCyl;

alpha1 = atan(abs(ACy)/abs(ACx));
alpha2 = atan(abs(ABy)/abs(ABx));

theta1 = acos( (abs(AB)^2 + abs(AC)^2 - (abs(BC))^2) / (2 * abs(AB) * abs(AC)) ) - alpha2 + alpha1;

thetaBoom = theta1;

== matlab function GreenCraneSimulator/PLC/MotionRefSelector/MATLAB Function ==
  data: AutoMode input; VelRef output; VelRefAuto input; PosRefAuto input; VelRefMan input; PosRef output; VFF output; PFC output
function [VelRef, PosRef, VFF, PFC] = fcn(AutoMode, VelRefAuto, PosRefAuto, VelRefMan)
if AutoMode == 1 
VelRef = VelRefAuto;
PosRef = PosRefAuto;
VFF = 1; 
PFC = 1; 
else 
VelRef = VelRefMan;
PosRef = 0.0;
VFF = 1; 
PFC = 0; 
end

== matlab function GreenCraneSimulator/Hydro-Mechanical System /Pressure Compensator1/Compensator From Morten Bak Paper ==
  data: p0 input; p_C output; p_S input; p_LS input
function p_C = fcn(p0, p_S, p_LS)

p_C = p_LS;

if p0 <= (p_S-p_LS)
p_C = p_LS+p0;
elseif 0<(p_S-p_LS) < p0
p_C = p_S - p_LS; 
elseif (p_S-p_LS) <= 0
    p_C = p_LS;
end

== matlab function GreenCraneSimulator/Hydro-Mechanical System /Directional Control Valve/Edge Openings/Edge P-A/MATLAB Function1 ==
  data: u_dcv input; u_PA output; OL_pa parameter; OL_pb parameter; UL_at parameter; UL_bt parameter
function u_PA = fcn(u_dcv,OL_pa, OL_pb, UL_at, UL_bt)

  u_PA = 0;

if OL_pa <=  u_dcv 
 u_PA = 0;
 
elseif u_dcv <  OL_pa
  u_PA= -(u_dcv-OL_pa)/(1+OL_pa);
end

== matlab function GreenCraneSimulator/Hydro-Mechanical System /Directional Control Valve/Edge Openings/Edge P-B/MATLAB Function1 ==
  data: u_dcv input; u_PB output; OL_pa parameter; OL_pb parameter; UL_at parameter; UL_bt parameter
function u_PB = fcn(u_dcv,OL_pa, OL_pb, UL_at, UL_bt)

  u_PB = 0;

if u_dcv <=   OL_pb
 u_PB = 0;
 
elseif  OL_pb < u_dcv 
  u_PB = (u_dcv-OL_pb)/(1-OL_pb);
end

== matlab function GreenCraneSimulator/Hydro-Mechanical System /Over-Centre Valve/Capasitance/Bulk Modulus/Effective Bulk Modulus/MATLAB Function ==
  data: p input; K_oil_eff output; patm parameter; eta_air parameter; kappa_air parameter; beta_F parameter
function K_oil_eff = fcn(p,patm, eta_air, kappa_air, beta_F)
p = p*1e5;
% Effective bulk modulus 
beta_eff_Pa  = 1/(1/beta_F+1/(((1-eta_air)*(patm/(p+patm))^(-1/kappa_air)/eta_air+1)*kappa_air*(p+patm)));
K_oil_eff = beta_eff_Pa*1e-5;

== matlab function GreenCraneSimulator/PLC/RampMotionProfileGenerator/RampSignal ==
  data: x0 input; v0 input; x_ref input; x output; v_ref input; t0 input; tRamp input; tWait input; v output; t input; T output; Error output
function [x,v,T, Error] = fcn(x0,v0, x_ref,v_ref,t0,tRamp,tWait,t)
x_SP = x_ref - x0;
vs=v_ref;
slopeExt=v0-vs;
slopeRetr=-vs-v0;

as = vs/tRamp;
s_acc=(vs^2-v0^2)/as;

tHold=(x_SP-s_acc)/vs;

if tHold < 0 
Error = 1;
else 
Error = 0;
end

t1=tRamp;
t2=tHold; 
t3=tRamp;
t4=tWait;
t5=t1;
t6=t2;
t7=t3;

x1 = x0 + v0*((t0+t1)-t0)-(slopeExt/t1)*((t0+t1)-t0)^2/2;
x2 = x1 + vs*((t0+t1+t2)-(t0+t1)); 
x4 = x_ref - v0*((t0+t1+t2+t3+t4+t5)-(t0+t1+t2+t3+t4))+(slopeRetr/t5)*((t0+t1+t2+t3+t4+t5)-(t0+t1+t2+t3+t4))^2/2; 
x5 = x4-vs*((t0+t1+t2+t3+t4+t5+t6)-(t0+t1+t2+t3+t4+t5));  

if Error == 1
x = x0;
v = v0; 
elseif t>=0 && t<t0
x = x0; 
v = v0;
elseif t>=t0 && t<(t0+t1)
x = x0 + v0*(t-t0)-(slopeExt/t1)*(t-t0)^2/2;
v = v0-(slopeExt/t1)*(t-t0);  
elseif t>=(t0+t1) && t<(t0+t1+t2)
x = x1 + vs*(t-(t0+t1)); 
v = vs; 
elseif t>=(t0+t1+t2) && t<(t0+t1+t2+t3)
x = x2+vs*(t-(t0+t1+t2))+(slopeExt/t3)*(t-(t0+t1+t2))^2/2; 
v = vs+(slopeExt/t3)*(t-(t0+t1+t2));   
elseif t>=(t0+t1+t2+t3) && t<(t0+t1+t2+t3+t4)
x = x_ref;
v = v0;  
elseif t>=(t0+t1+t2+t3+t4) && t<(t0+t1+t2+t3+t4+t5)
x = x_ref - v0*(t-(t0+t1+t2+t3+t4))+(slopeRetr/t5)*(t-(t0+t1+t2+t3+t4))^2/2; 
v = v0+(slopeRetr/t5)*(t-(t0+t1+t2+t3+t4));     
elseif t>=(t0+t1+t2+t3+t4+t5) && t<(t0+t1+t2+t3+t4+t5+t6)
x = x4-vs*(t-(t0+t1+t2+t3+t4+t5));   
v = -vs;    
elseif t>=(t0+t1+t2+t3+t4+t5+t6) && t<(t0+t1+t2+t3+t4+t5+t6+t7)
x = x5-vs*(t-(t0+t1+t2+t3+t4+t5+t6))-(slopeRetr/t3)*(t-(t0+t1+t2+t3+t4+t5+t6))^2/2;    
v = -vs-(slopeRetr/t3)*(t-(t0+t1+t2+t3+t4+t5+t6));     
else 
x = x0;
v = v0; 
end

T = t0+t1+t2+t3+t4+t5+t6+t7;

== matlab function GreenCraneSimulator/Hydro-Mechanical System /Rigid Mechanical System - Green Crane Arm/Lasse Schmidt ==
  data: Geq output; Ceq output; Meq output; x input

function [Geq,Ceq, Meq]  = fcn(x)

% Mechanical Model Green Crane @ UiA Laboratory 

% Parameters 
L_AGx = 3139/1000;            % [m]
L_AGy = 64*(1/1000);          % [m]
L_ACx = 550*(1/1000);         % [m]
L_ACy = 130*(1/1000);         % [m]
L_ABx = 420*(1/1000);         % [m]
L_ABy = 1055*(1/1000);        % [m]
L_AB = sqrt(L_ABx^2+L_ABy^2); % [m]
L_AC = sqrt(L_ACx^2+L_ACy^2); % [m]
L_AG = sqrt(L_AGx^2+L_AGy^2); % [m]
m_cm = 402;                   % [kg]
J_A = 4251.2;                 % [kg*m^2]
J_cm = J_A-L_AG^2*m_cm;       % [kg*m^2]
L_min = 772*(1/1000);         % [m]
g = 9.82;                     % [m/s^2]

% Gravitational Load [N]
Geq = -0.2e1*sqrt(-(x-L_AB+L_min+L_AC)*(x+L_min-L_AC-L_AB)*(x+L_AB+L_min-L_AC)*(x+L_AB+L_min+L_AC))*g*m_cm*(cos(acos((L_AB^2+L_AC^2-(x+L_min)^2)/L_AC/L_AB/0.2e1)-atan(L_ABy/L_ABx)+atan(L_ACy/L_ACx)+atan(L_AGy/L_AGx))*L_AGx-sin(acos((L_AB^2+L_AC^2-(x+L_min)^2)/L_AC/L_AB/0.2e1)-atan(L_ABy/L_ABx)+atan(L_ACy/L_ACx)+atan(L_AGy/L_AGx))*L_AGy)*(x+L_min)/(x-L_AB+L_min+L_AC)/(x+L_min-L_AC-L_AB)/(x+L_AB+L_min-L_AC)/(x+L_AB+L_min+L_AC);

% Equalent Inertial Load [kg]
Meq = -4*(L_AGx^2*(x+L_min)*m_cm+L_AGy^2*(x+L_min)*m_cm+(x+L_min)*J_cm)*(x+L_min)/(-x+L_AB-L_min-L_AC)/(-x+L_AB-L_min+L_AC)/(x+L_AB+L_min+L_AC)/(x+L_AB+L_min-L_AC);

% Coriolis Force [N*(m/s)^2]
Ceq = 4*((L_AGx^2+L_AGy^2)*m_cm+J_cm)*(x+L_min)*(-L_AB^2+L_AC^2+(x+L_min)^2)*(L_AB^2-L_AC^2+(x+L_min)^2)/(x+L_min-L_AC-L_AB)^2/(x-L_AB+L_min+L_AC)^2/(x+L_AB+L_min+L_AC)^2/(x+L_AB+L_min-L_AC)^2;

== matlab function GreenCraneSimulator/Hydro-Mechanical System /Subsystem/CH Bore Side/Bulk Modulus/Effective Bulk Modulus/MATLAB Function ==
  data: p input; K_oil_eff output; patm parameter; eta_air parameter; kappa_air parameter; beta_F parameter
function K_oil_eff = fcn(p,patm, eta_air, kappa_air, beta_F)
p = p*1e5;
% Effective bulk modulus 
beta_eff_Pa  = 1/(1/beta_F+1/(((1-eta_air)*(patm/(p+patm))^(-1/kappa_air)/eta_air+1)*kappa_air*(p+patm)));
K_oil_eff = beta_eff_Pa*1e-5;

== matlab function GreenCraneSimulator/Hydro-Mechanical System /Subsystem/CH Rod Side/Bulk Modulus/Effective Bulk Modulus/MATLAB Function ==
  data: p input; K_oil_eff output; patm parameter; eta_air parameter; kappa_air parameter; beta_F parameter
function K_oil_eff = fcn(p,patm, eta_air, kappa_air, beta_F)
p = p*1e5;
% Effective bulk modulus 
beta_eff_Pa  = 1/(1/beta_F+1/(((1-eta_air)*(patm/(p+patm))^(-1/kappa_air)/eta_air+1)*kappa_air*(p+patm)));
K_oil_eff = beta_eff_Pa*1e-5;
